simulink model "gle"  (R2015b)
settings: Solver=FixedStepDiscrete  StartTime=0.0  StopTime=params.stop_time  FixedStep=params.sample_time  RelTol=1e-3
values from neighbouring files (symbols this model uses):
  params = calculate_sim_params(k_B, N_steps, T, mass, A)    [plot_average_isf.m]    (also in plot_band_pass_trajectory.m = calculate_sim_params(k_B, N, T, mass, A); plot_delta_like_trajectory.m = calculate_sim_params(k_B, N, T, mass, A); plot_function_delta_comb_trajectory.m = calculate_sim_params(k_B, N, T, mass, A); plot_low_pass_3d_trajectory.m = calculate_sim_params(k_B, N, T, mass, A))
undefined symbols (not defined in the file or in its folder): DiscIntNeverNeededParam
libraries: simulink x1
settings Model: Creator=rlc61  LastModifiedBy=Ryan
settings DataIOCC: SaveFormat=Array
settings DebuggingCC: SolverPrmCheckMsg=warning
settings HardwareCC: ProdBitPerPointer=32  ProdLargestAtomicFloat=None  ProdIntDivRoundTo=Undefined  ProdEndianess=Unspecified  ProdWordSize=32  ProdHWDeviceType=32-bit Generic
settings GRTTargetCC: GeneratePreprocessorConditionals=Disable all
settings ConfigComp: CovModelRefEnable=Off  CovSFcnEnable=off

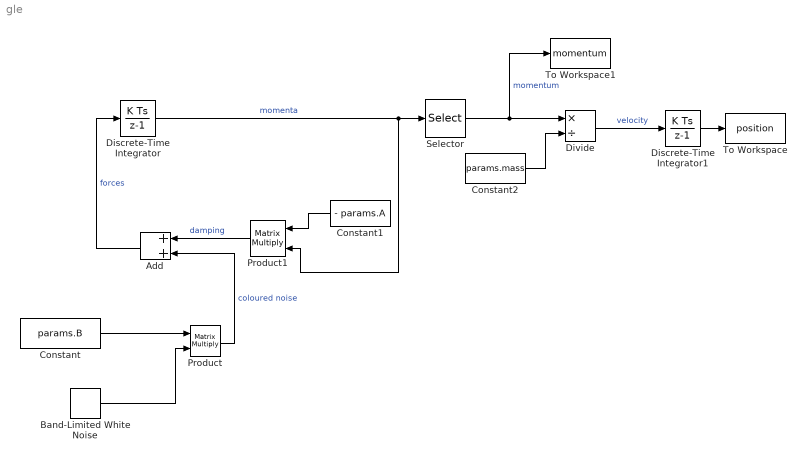
== system gle ==
  Add : Sum
  Band-Limited White Noise : simulink/Sources/Band-Limited White Noise  Cov=params.psd  Ts=params.sample_time  seed=params.seed_values
  Constant : Constant  Value=params.B
  Constant1 : Constant  Value=- params.A
  Constant2 : Constant  Value=params.mass
  Discrete-Time Integrator : DiscreteIntegrator  InitialCondition=params.p_init  InitialConditionSetting=State (most efficient)  SampleTime=params.sample_time  ICPrevOutput=DiscIntNeverNeededParam  ICPrevScaledInput=DiscIntNeverNeededParam
  Discrete-Time Integrator1 : DiscreteIntegrator  InitialCondition=params.r_init  InitialConditionSetting=State (most efficient)  SampleTime=params.sample_time  ICPrevOutput=DiscIntNeverNeededParam  ICPrevScaledInput=DiscIntNeverNeededParam
  Divide : Product  Inputs=*/
  Product : Product  Multiplication=Matrix(*)
  Product1 : Product  Multiplication=Matrix(*)
  Selector : Selector  IndexOptions=Index vector (dialog)  Indices=1  OutputSizes=1
  To Workspace : ToWorkspace  VariableName=position  SaveFormat=Timeseries  SampleTime=-1
      settings: MaxDataPoints=params.last_position  Decimation=params.decimation
  To Workspace1 : ToWorkspace  VariableName=momentum  SaveFormat=Timeseries  SampleTime=-1
      settings: MaxDataPoints=params.last_momenta  Decimation=params.decimation
  wires:
  Add/1 -> Discrete-Time Integrator/1  "forces"
  Product1/1 -> Add/1  "damping"
  Divide/1 -> Discrete-Time Integrator1/1  "velocity"
  Discrete-Time Integrator1/1 -> To Workspace/1
  Constant/1 -> Product/1
  Band-Limited White Noise/1 -> Product/2
  Constant1/1 -> Product1/1
  Constant2/1 -> Divide/2
  Discrete-Time Integrator/1 -> Selector/1, Product1/2  "momenta"
  Selector/1 -> To Workspace1/1, Divide/1  "momentum"
  Product/1 -> Add/2  "coloured noise"
